simulink model "P2"  (R2025b)
settings: Solver=FixedStepAuto  StartTime=0.0  StopTime=0.1  FixedStep=1e-6
values from neighbouring files (symbols this model uses):
  C = 2.56e-3    (= 0.00256)    [P4.m]    (also in Proiect3_1.m = 0.00078125; ProiectEP_3.m = 0.00078125; ProiectEP_Init.m = 0.00078125; Proiect_2.m = 0.00078125)
  f = 1500    [P4.m]    (also in Proiect3_1.m; ProiectEP_3.m; ProiectEP_Init.m; Proiect_2.m)
  L = 2.944e-3    (= 0.002944)    [P4.m]    (also in Proiect3_1.m = 0.001405155; ProiectEP_3.m = 0.001405155; ProiectEP_Init.m = 0.001405155; Proiect_2.m = 0.001405155)
  miu = 0.20833    [P4.m]    (also in Proiect3_1.m = 0.208; ProiectEP_3.m = 0.208; ProiectEP_Init.m = 0.208; Proiect_2.m)
  R = 0.1    [P4.m]    (also in Proiect3_1.m = 0.4; ProiectEP_3.m = 0.4; ProiectEP_Init.m = 0.4; Proiect_2.m = 0.4)
  Uin = 48    [P4.m]    (also in Proiect3_1.m; ProiectEP_3.m; ProiectEP_Init.m; Proiect_2.m)
settings Model: Creator=Razvan  LastModifiedBy=Razvan

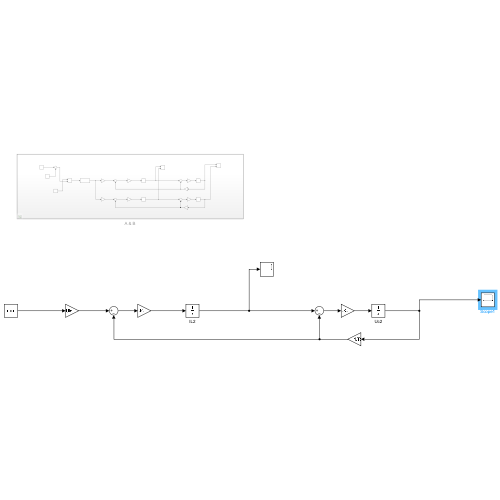
[thumbnail: Simulink's stored preview of the top-level diagram]
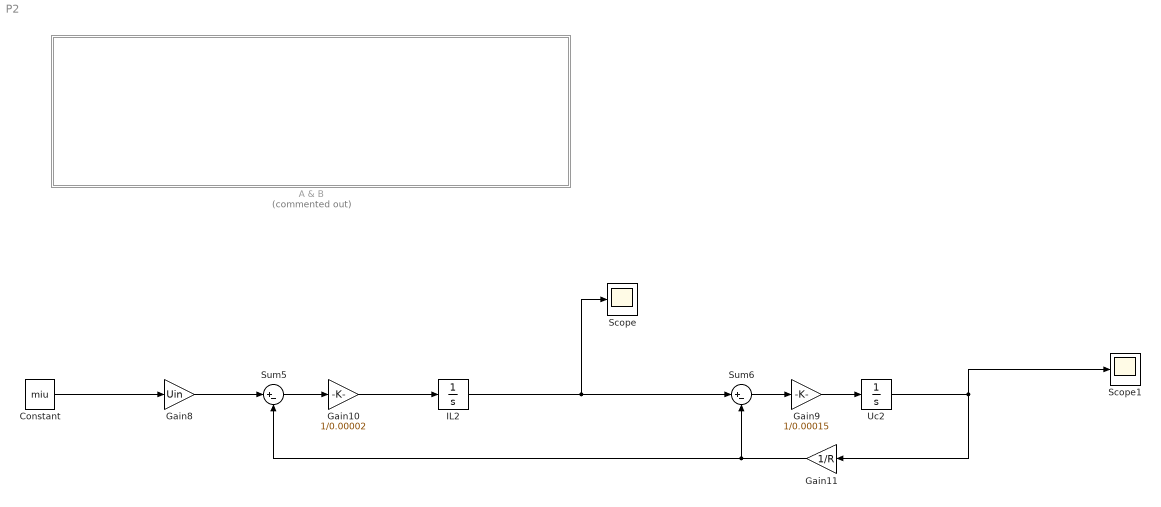
== system P2 ==
  A & B : Subsystem  Commented=on
  Constant : Constant  Value=miu
  Gain10 : Gain  Gain=1/0.00002
  Gain11 : Gain  Gain=1/R
  Gain8 : Gain  Gain=Uin
  Gain9 : Gain  Gain=1/0.00015
  IL2 : Integrator
  Scope : Scope
      settings: ActiveDisplayYMinimum=-50.989683712952235  ActiveDisplayYMaximum=47.454950726909068  DataLoggingVariableName=ScopeData2
  Scope1 : Scope
      settings: ActiveDisplayYMinimum=-0.13855164502221973  ActiveDisplayYMaximum=1.2469648051999778  DataLoggingVariableName=ScopeData3
  Sum5 : Sum  Inputs=|+-
  Sum6 : Sum  Inputs=|+-
  Uc2 : Integrator
  wires:
  Gain9/1 -> Uc2/1
  IL2/1 -> Scope/1, Sum6/1
  Gain8/1 -> Sum5/1
  Sum5/1 -> Gain10/1
  Gain10/1 -> IL2/1
  Uc2/1 -> Gain11/1, Scope1/1
  Gain11/1 -> Sum5/2, Sum6/2
  Sum6/1 -> Gain9/1
  Constant/1 -> Gain8/1

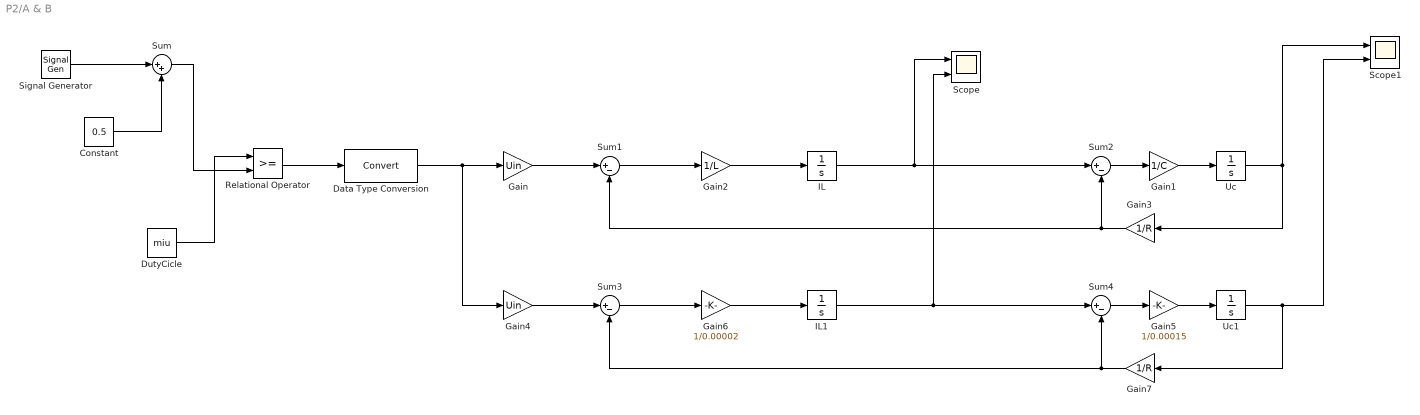
== system P2/A & B ==
  Constant : Constant  Value=0.5
  Data Type Conversion : DataTypeConversion  SaturateOnIntegerOverflow=off  RndMeth=Floor
  DutyCicle : Constant  Value=miu
  Gain : Gain  Gain=Uin
  Gain1 : Gain  Gain=1/C
  Gain2 : Gain  Gain=1/L
  Gain3 : Gain  Gain=1/R
  Gain4 : Gain  Gain=Uin
  Gain5 : Gain  Gain=1/0.00015
  Gain6 : Gain  Gain=1/0.00002
  Gain7 : Gain  Gain=1/R
  IL : Integrator
  IL1 : Integrator
  Relational Operator : RelationalOperator  OutDataTypeStr=boolean  RndMeth=Simplest  InputSameDT=off
  Scope : Scope  NumInputPorts=2
      settings: ActiveDisplayYMinimum=-15.395401396076515  ActiveDisplayYMaximum=63.647422758570059
  Scope1 : Scope  NumInputPorts=2
      settings: ActiveDisplayYMinimum=-1.2289289077672709  ActiveDisplayYMaximum=7.689852053591018
  Signal Generator : SignalGenerator  WaveForm=sawtooth  Amplitude=0.5  Frequency=f
  Sum : Sum  Inputs=|++
  Sum{1..4} (4 alike) : Sum  Inputs=|+-
  Uc : Integrator
  Uc1 : Integrator
  wires:
  Gain6/1 -> IL1/1
  Gain1/1 -> Uc/1
  Gain/1 -> Sum1/1
  IL1/1 -> Scope/2, Sum4/1
  IL/1 -> Scope/1, Sum2/1
  Sum1/1 -> Gain2/1
  Signal Generator/1 -> Sum/1
  Data Type Conversion/1 -> Gain4/1, Gain/1
  Sum2/1 -> Gain1/1
  Gain3/1 -> Sum1/2, Sum2/2
  Relational Operator/1 -> Data Type Conversion/1
  Sum3/1 -> Gain6/1
  Constant/1 -> Sum/2
  Uc/1 -> Gain3/1, Scope1/1
  Gain2/1 -> IL/1
  Gain7/1 -> Sum3/2, Sum4/2
  DutyCicle/1 -> Relational Operator/1
  Sum/1 -> Relational Operator/2
  Sum4/1 -> Gain5/1
  Uc1/1 -> Scope1/2, Gain7/1
  Gain4/1 -> Sum3/1
  Gain5/1 -> Uc1/1
